simulink model "Ecotron"  (R2019b)
settings: Solver=FixedStepAuto  StartTime=0.0  StopTime=1  FixedStep=0.001  RelTol=1e-3  EnableMultiTasking=on
InitFcn:
  | EcoCoder_PreCheckLic();
libraries: CoderSF_BSW_Libs x228, SF_CanService_Libs x49, simulink x33, dspstat3 x6
(part 2 of 6)

== system Ecotron/Input/By-wire/Throttle Controller ==
  Bus Creator : BusCreator  Inputs=4
  Bus Creator1 : BusCreator  Inputs=4  OutDataTypeStr=Bus: Msg
      settings: InheritFromInputs=off
  Read CAN Message : SF_CanService_Libs/Read CAN Message  typeCAN=Connected  channel=CAN_C  mEn=off  msgInfo=Leo_accpedal  msgItermStore=Feedback  msgIterm=Feedback  valid=on  stale=on  motoBit=off  setSignalName=on  flgCustomMonitorVariableRules=on  defineSignalName=off  prefixSignal='rx'  flgValTest=off  flgNoFixed=on  tSample=Task_L1ms  modeCode=Parameterless
  Subsystem4 : Subsystem
  Write and Read Measurement : CoderSF_BSW_Libs/Calibration & Measurement/Write and Read Measurement  variable_name=THROTTLE_CurrentPedalPos  variable_value=0  variable_type=single  numD=1  unitStr=""  descStr=""
      settings: AttributesFormatString=type:%<variable_type> Dimensions:%<numD>  SourceProductName=EcoCoder Blocks
  Write and Read Measurement1 : CoderSF_BSW_Libs/Calibration & Measurement/Write and Read Measurement  variable_name=THROTTLE_ECUTimeout  variable_value=0  variable_type=single  numD=1  unitStr=""  descStr=""
      settings: AttributesFormatString=type:%<variable_type> Dimensions:%<numD>  SourceProductName=EcoCoder Blocks
  Write and Read Measurement2 : CoderSF_BSW_Libs/Calibration & Measurement/Write and Read Measurement  variable_name=THROTTLE_PedalConnectionError  variable_value=0  variable_type=single  numD=1  unitStr=""  descStr=""
      settings: AttributesFormatString=type:%<variable_type> Dimensions:%<numD>  SourceProductName=EcoCoder Blocks
  Throttle : Outport
  wires:
  Bus Creator/1 -> Throttle/1
  Read CAN Message/4 -> Write and Read Measurement1/1  "rxTimeout_Err"
  Read CAN Message/5 -> Write and Read Measurement2/1  "rxPedal_connErr"
  Subsystem4/2(Cnt) -> Bus Creator1/2  "Cnt"
  Subsystem4/4(Msg_Freq) -> Bus Creator1/4  "MsgFreq"
  Subsystem4/3(Timeout_Err) -> Bus Creator1/3  "Timeout"
  Subsystem4/1("Available ") -> Bus Creator1/1  "Available"
  Read CAN Message/1 -> Subsystem4/1("Available_in ")
  Read CAN Message/2 -> Subsystem4/2(Msg_cnt)
  Bus Creator1/1 -> Bus Creator/1  "Msg"
  Read CAN Message/3 -> Write and Read Measurement/1  "rxCurrent_PedalPos"
  Write and Read Measurement/1 -> Bus Creator/2  "THROTTLE_CurrentPedalPos"
  Write and Read Measurement1/1 -> Bus Creator/3  "THROTTLE_ECUTimeout"
  Write and Read Measurement2/1 -> Bus Creator/4  "THROTTLE_PedalConnectionError"

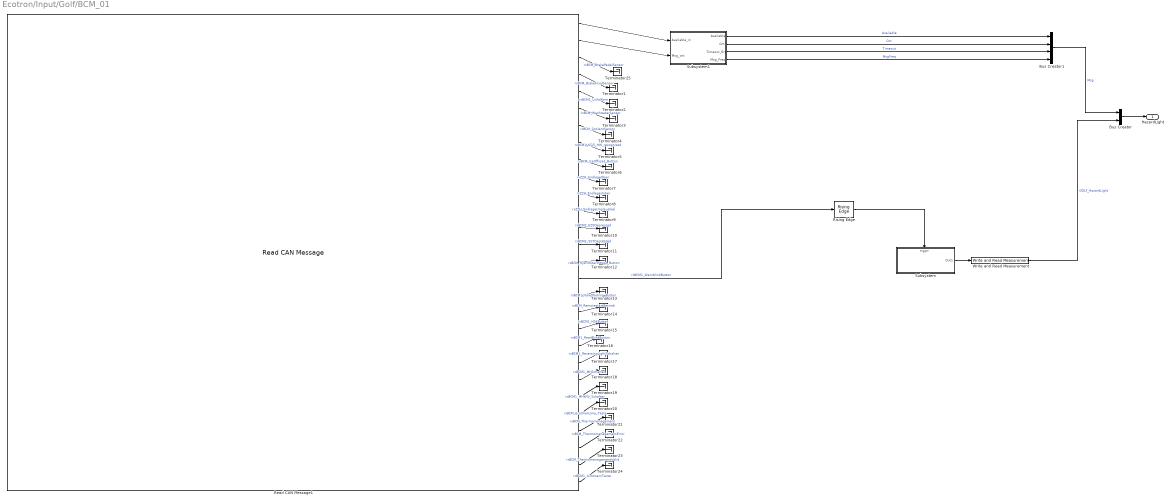
== system Ecotron/Input/Golf/BCM_01 ==
  Bus Creator : BusCreator  Inputs=2
  Bus Creator1 : BusCreator  Inputs=4  OutDataTypeStr=Bus: Msg
      settings: InheritFromInputs=off
  Read CAN Message1 : SF_CanService_Libs/Read CAN Message  typeCAN=Connected  channel=CAN_B  mEn=off  msgInfo=vw_golf  msgItermStore=BCM_01  msgIterm=BCM_01  valid=on  stale=on  motoBit=off  setSignalName=on  flgCustomMonitorVariableRules=on  defineSignalName=off  prefixSignal='rx'  flgValTest=off  flgNoFixed=on  tSample=Task_L1ms  modeCode=Parameterless
  Rising Edge : CoderSF_BSW_Libs/Application Base Blocks/Rising Edge  InitialCondition=off
      settings: SourceProductName=EcoCoder Blocks
  Subsystem : Subsystem
  Subsystem1 : Subsystem
  Terminator{1..25} (25 alike) : Terminator
  Write and Read Measurement : CoderSF_BSW_Libs/Calibration & Measurement/Write and Read Measurement  variable_name=GOLF_HazardLight  variable_value=0  variable_type=boolean  numD=1  unitStr=""  descStr=""
      settings: AttributesFormatString=type:%<variable_type> Dimensions:%<numD>  SourceProductName=EcoCoder Blocks
  HazardLight : Outport
  wires:
  Read CAN Message1/7 -> Terminator4/1  "rxBCM_CoolantSensor"
  Read CAN Message1/25 -> Terminator21/1  "rxBCM_Thermomanagement"
  Read CAN Message1/3 -> Terminator25/1  "rxBCM_BrakePedalSensor"
  Read CAN Message1/5 -> Terminator2/1  "rxBCM1_LichtWarn"
  Read CAN Message1/20 -> Terminator16/1  "rxBCM1_RearBlindButton"
  Read CAN Message1/4 -> Terminator1/1  "rxBCM_BrakeFluidSensor"
  Read CAN Message1/12 -> Terminator9/1  "rxZZH_EndlageUnplausibel"
  Read CAN Message1/11 -> Terminator8/1  "rxZZH_EndlageUnten"
  Read CAN Message1/9 -> Terminator6/1  "rxBCM_IceOffroad_Button"
  Read CAN Message1/28 -> Terminator24/1  "rxBCM1_LichtwarnTexte"
  Read CAN Message1/8 -> Terminator5/1  "rxBCM1_Kl15_HW_recognized"
  Read CAN Message1/6 -> Terminator3/1  "rxBCM_WashwaterSensor"
  Read CAN Message1/24 -> Terminator20/1  "rxBCM_EcoCharisma_Taste"
  Read CAN Message1/10 -> Terminator7/1  "rxZZH_EndlageOben"
  Read CAN Message1/14 -> Terminator11/1  "rxBCM2_SSTDepressed"
  Read CAN Message1/13 -> Terminator10/1  "rxBCM2_EZSDepressed"
  Read CAN Message1/15 -> Terminator12/1  "rxBCM_HybridStartStopp_Button"
  Read CAN Message1/17 -> Terminator13/1  "rxBCM1_ValetParking_Button"
  Read CAN Message1/18 -> Terminator14/1  "rxBCM_RemotestartBetrieb"
  Read CAN Message1/16 -> Rising Edge/1  "rxBCM1_WarnblinkButton"
  Read CAN Message1/22 -> Terminator18/1  "rxBCM1_MHSchalter"
  Read CAN Message1/19 -> Terminator15/1  "rxBCM1_HSKButton"
  Read CAN Message1/23 -> Terminator19/1  "rxBCM1_MHWIV_Schalter"
  Read CAN Message1/21 -> Terminator17/1  "rxBCM1_ReversingLightSchalter"
  Read CAN Message1/26 -> Terminator22/1  "rxBCM_ThermomanagementError"
  Read CAN Message1/27 -> Terminator23/1  "rxBCM_ThermomanagementValid"
  Subsystem1/2(Cnt) -> Bus Creator1/2  "Cnt"
  Subsystem1/1("Available ") -> Bus Creator1/1  "Available"
  Read CAN Message1/2 -> Subsystem1/2(Msg_cnt)
  Subsystem1/4(Msg_Freq) -> Bus Creator1/4  "MsgFreq"
  Bus Creator1/1 -> Bus Creator/1  "Msg"
  Read CAN Message1/1 -> Subsystem1/1("Available_in ")
  Subsystem1/3(Timeout_Err) -> Bus Creator1/3  "Timeout"
  Subsystem/1(Out1) -> Write and Read Measurement/1
  Rising Edge/1 -> Subsystem/Trigger
  Write and Read Measurement/1 -> Bus Creator/2  "GOLF_HazardLight"
  Bus Creator/1 -> HazardLight/1

== system Ecotron/Input/Golf/Brake ==
  Bus Creator : BusCreator  Inputs=2
  Bus Creator1 : BusCreator  Inputs=4  OutDataTypeStr=Bus: Msg
      settings: InheritFromInputs=off
  Read CAN Message : SF_CanService_Libs/Read CAN Message  typeCAN=Connected  channel=CAN_B  mEn=off  msgInfo=vw_golf  msgItermStore=Brake  msgIterm=Brake  valid=on  stale=on  motoBit=off  setSignalName=on  flgCustomMonitorVariableRules=on  defineSignalName=off  prefixSignal=''  flgValTest=off  flgNoFixed=on  tSample=Task_L1ms  modeCode=Parameterless
  Subsystem1 : Subsystem
  Write and Read Measurement : CoderSF_BSW_Libs/Calibration & Measurement/Write and Read Measurement  variable_name=GOLF_BrakePedalPos  variable_value=0  variable_type=single  numD=1  unitStr=""  descStr=""
      settings: AttributesFormatString=type:%<variable_type> Dimensions:%<numD>  SourceProductName=EcoCoder Blocks
  Brake : Outport
  wires:
  Subsystem1/2(Cnt) -> Bus Creator1/2  "Cnt"
  Subsystem1/4(Msg_Freq) -> Bus Creator1/4  "MsgFreq"
  Subsystem1/3(Timeout_Err) -> Bus Creator1/3  "Timeout"
  Subsystem1/1("Available ") -> Bus Creator1/1  "Available"
  Read CAN Message/1 -> Subsystem1/1("Available_in ")
  Read CAN Message/2 -> Subsystem1/2(Msg_cnt)
  Bus Creator1/1 -> Bus Creator/1  "Msg"
  Read CAN Message/3 -> Write and Read Measurement/1  "Brake_pedalPos"
  Bus Creator/1 -> Brake/1  "Brake"
  Write and Read Measurement/1 -> Bus Creator/2  "GOLF_BrakePedalPos"

== system Ecotron/Input/Golf/Brake and Steering Feedback Echo ==
  Receive CAN Message : CoderSF_BSW_Libs/CAN/Receive CAN Message  channel=CAN_B  txid=hex2dec('176')  extended=off  txlen=8  tasktimeIndex=Task_L1ms
      settings: SourceProductName=EcoCoder Blocks
  Receive CAN Message1 : CoderSF_BSW_Libs/CAN/Receive CAN Message  channel=CAN_B  txid=hex2dec('86')  extended=off  txlen=8  tasktimeIndex=Task_L1ms
      settings: SourceProductName=EcoCoder Blocks
  Subsystem2 : Subsystem
  Subsystem7 : Subsystem
  Terminator{2..9} (8 alike) : Terminator
  wires:
  Receive CAN Message/4 -> Terminator5/1
  Receive CAN Message1/3 -> Terminator8/1
  Receive CAN Message1/4 -> Terminator3/1
  Receive CAN Message/6 -> Subsystem2/1(In1)
  Receive CAN Message1/5 -> Terminator2/1
  Receive CAN Message1/2 -> Terminator9/1
  Receive CAN Message/3 -> Terminator6/1
  Receive CAN Message1/6 -> Subsystem7/1(In1)
  Receive CAN Message1/1 -> Subsystem7/Trigger
  Receive CAN Message/5 -> Terminator4/1
  Receive CAN Message/1 -> Subsystem2/Trigger
  Receive CAN Message/2 -> Terminator7/1

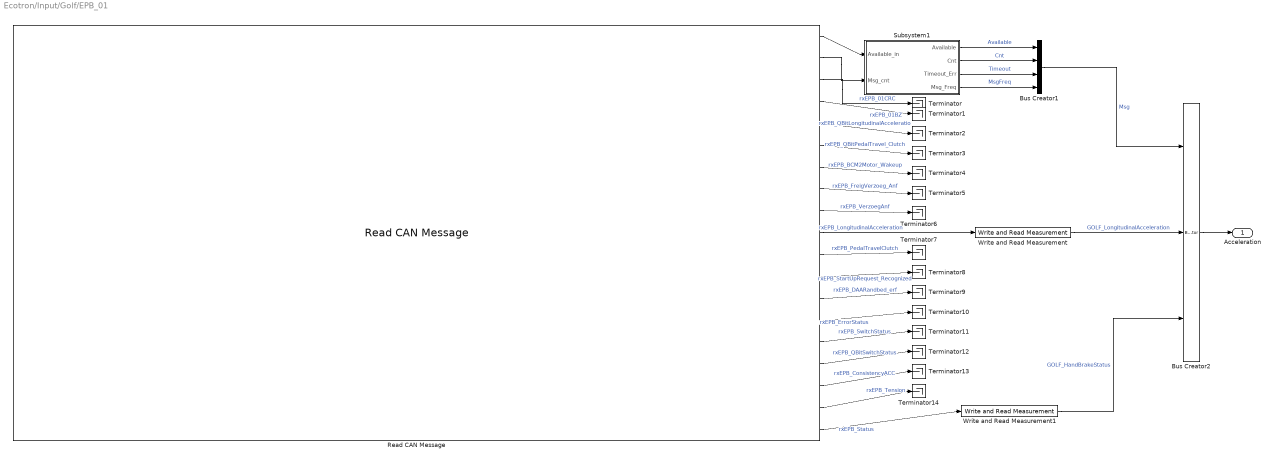
== system Ecotron/Input/Golf/EPB_01 ==
  Bus Creator1 : BusCreator  Inputs=4  OutDataTypeStr=Bus: Msg
      settings: InheritFromInputs=off
  Bus Creator2 : BusCreator  Inputs=3
  Read CAN Message : SF_CanService_Libs/Read CAN Message  typeCAN=Connected  channel=CAN_B  mEn=off  msgInfo=vw_golf  msgItermStore=EPB_01  msgIterm=EPB_01  valid=on  stale=on  motoBit=off  setSignalName=on  flgCustomMonitorVariableRules=on  defineSignalName=off  prefixSignal='rx'  flgValTest=off  flgNoFixed=on  tSample=Task_L1ms  modeCode=Parameterless
  Subsystem1 : Subsystem
  Terminator{,1..14} (15 alike) : Terminator
  Write and Read Measurement : CoderSF_BSW_Libs/Calibration & Measurement/Write and Read Measurement  variable_name=GOLF_LongitudinalAcceleration  variable_value=0  variable_type=single  numD=1  unitStr=""  descStr=""
      settings: AttributesFormatString=type:%<variable_type> Dimensions:%<numD>  SourceProductName=EcoCoder Blocks
  Write and Read Measurement1 : CoderSF_BSW_Libs/Calibration & Measurement/Write and Read Measurement  variable_name=GOLF_HandBrakeStatus  variable_value=0  variable_type=single  numD=1  unitStr=""  descStr=""
      settings: AttributesFormatString=type:%<variable_type> Dimensions:%<numD>  SourceProductName=EcoCoder Blocks
  Acceleration : Outport
  wires:
  Read CAN Message/8 -> Terminator5/1  "rxEPB_FreigVerzoeg_Anf"
  Read CAN Message/6 -> Terminator3/1  "rxEPB_QBitPedalTravel_Clutch"
  Subsystem1/2(Cnt) -> Bus Creator1/2  "Cnt"
  Subsystem1/1("Available ") -> Bus Creator1/1  "Available"
  Read CAN Message/19 -> Write and Read Measurement1/1  "rxEPB_Status"
  Read CAN Message/3 -> Terminator/1  "rxEPB_01CRC"
  Read CAN Message/2 -> Subsystem1/2(Msg_cnt)
  Read CAN Message/11 -> Terminator7/1  "rxEPB_PedalTravelClutch"
  Read CAN Message/16 -> Terminator12/1  "rxEPB_QBitSwitchStatus"
  Read CAN Message/7 -> Terminator4/1  "rxEPB_BCM2Motor_Wakeup"
  Read CAN Message/14 -> Terminator10/1  "rxEPB_ErrorStatus"
  Read CAN Message/9 -> Terminator6/1  "rxEPB_VerzoegAnf"
  Subsystem1/4(Msg_Freq) -> Bus Creator1/4  "MsgFreq"
  Read CAN Message/15 -> Terminator11/1  "rxEPB_SwitchStatus"
  Subsystem1/3(Timeout_Err) -> Bus Creator1/3  "Timeout"
  Read CAN Message/13 -> Terminator9/1  "rxEPB_DAARandbed_erf"
  Read CAN Message/4 -> Terminator1/1  "rxEPB_01BZ"
  Read CAN Message/10 -> Write and Read Measurement/1  "rxEPB_LongitudinalAcceleration"
  Read CAN Message/18 -> Terminator14/1  "rxEPB_Tension"
  Read CAN Message/5 -> Terminator2/1  "rxEPB_QBitLongitudinalAcceleratio"
  Read CAN Message/12 -> Terminator8/1  "rxEPB_StartUpRequest_Recognized"
  Read CAN Message/1 -> Subsystem1/1("Available_in ")
  Bus Creator1/1 -> Bus Creator2/1  "Msg"
  Read CAN Message/17 -> Terminator13/1  "rxEPB_ConsistencyACC"
  Bus Creator2/1 -> Acceleration/1
  Write and Read Measurement/1 -> Bus Creator2/2  "GOLF_LongitudinalAcceleration"
  Write and Read Measurement1/1 -> Bus Creator2/3  "GOLF_HandBrakeStatus"

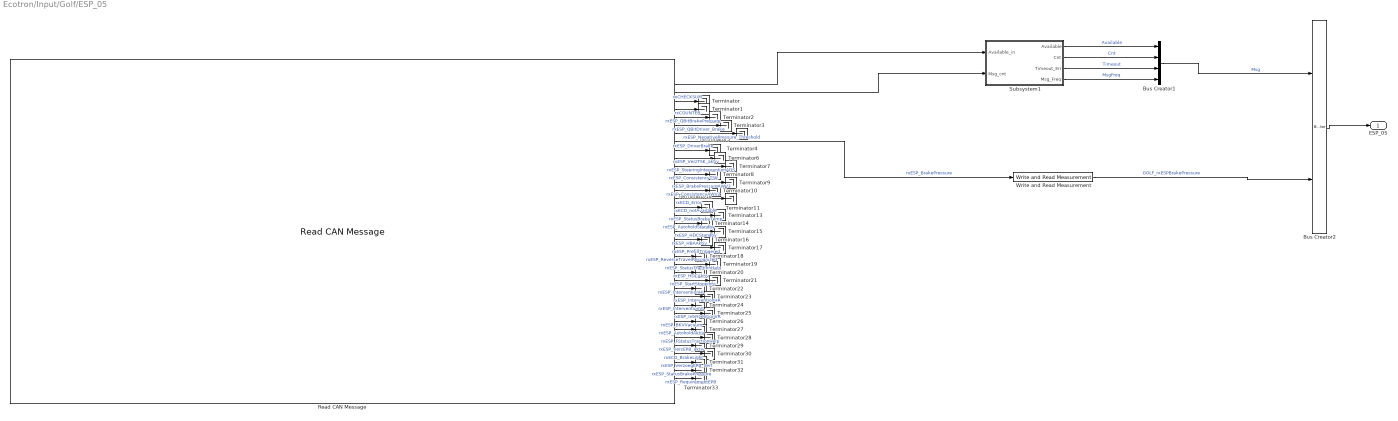
== system Ecotron/Input/Golf/ESP_05 ==
  Bus Creator1 : BusCreator  Inputs=4  OutDataTypeStr=Bus: Msg
      settings: InheritFromInputs=off
  Bus Creator2 : BusCreator  Inputs=2
  Read CAN Message : SF_CanService_Libs/Read CAN Message  typeCAN=Connected  channel=CAN_B  mEn=off  msgInfo=vw_golf  msgItermStore=ESP_05  msgIterm=ESP_05  valid=on  stale=on  motoBit=off  setSignalName=on  flgCustomMonitorVariableRules=on  defineSignalName=off  prefixSignal='rx'  flgValTest=off  flgNoFixed=on  tSample=Task_L1ms  modeCode=Parameterless
  Subsystem1 : Subsystem
  Terminator{,1..33} (34 alike) : Terminator
  Write and Read Measurement : CoderSF_BSW_Libs/Calibration & Measurement/Write and Read Measurement  variable_name=GOLF_rxESPBrakePressure  variable_value=0  variable_type=single  numD=1  unitStr=""  descStr=""
      settings: AttributesFormatString=type:%<variable_type> Dimensions:%<numD>  SourceProductName=EcoCoder Blocks
  ESP_05 : Outport
  wires:
  Subsystem1/1("Available ") -> Bus Creator1/1  "Available"
  Bus Creator2/1 -> ESP_05/1
  Read CAN Message/2 -> Subsystem1/2(Msg_cnt)
  Subsystem1/2(Cnt) -> Bus Creator1/2  "Cnt"
  Read CAN Message/1 -> Subsystem1/1("Available_in ")
  Subsystem1/3(Timeout_Err) -> Bus Creator1/3  "Timeout"
  Bus Creator1/1 -> Bus Creator2/1  "Msg"
  Subsystem1/4(Msg_Freq) -> Bus Creator1/4  "MsgFreq"
  Write and Read Measurement/1 -> Bus Creator2/2  "GOLF_rxESPBrakePressure"
  Read CAN Message/8 -> Write and Read Measurement/1  "rxESP_BrakePressure"
  Read CAN Message/3 -> Terminator/1  "rxCHECKSUM"
  Read CAN Message/4 -> Terminator1/1  "rxCOUNTER"
  Read CAN Message/5 -> Terminator2/1  "rxESP_QBitBrakePressure"
  Read CAN Message/6 -> Terminator3/1  "rxESP_QBitDriver_Brake"
  Read CAN Message/7 -> Terminator4/1  "rxESP_NegativePressure_Threshold"
  Read CAN Message/9 -> Terminator5/1  "rxESP_DriverBrake"
  Read CAN Message/10 -> Terminator6/1  "rxESP_VerzTSK_aktiv"
  Read CAN Message/11 -> Terminator7/1  "rxESP_SteeringInterventionADS"
  Read CAN Message/12 -> Terminator8/1  "rxESP_ConsistencyTSK"
  Read CAN Message/13 -> Terminator9/1  "rxESP_BrakePressureAWV2"
  Read CAN Message/14 -> Terminator10/1  "rxESP_ConsistencyAWV2"
  Read CAN Message/15 -> Terminator11/1  "rxECD_Error"
  Read CAN Message/16 -> Terminator12/1  "rxECD_notAvailable"
  Read CAN Message/17 -> Terminator13/1  "rxESP_StatusBrakeTemp"
  Read CAN Message/18 -> Terminator14/1  "rxESP_AutoholdStandby"
  Read CAN Message/19 -> Terminator15/1  "rxESP_HDCStandby"
  Read CAN Message/20 -> Terminator16/1  "rxESP_HBAAktiv"
  Read CAN Message/21 -> Terminator17/1  "rxESP_PrefillTriggered"
  Read CAN Message/22 -> Terminator18/1  "rxESP_ReverseTravelRecognized"
  Read CAN Message/23 -> Terminator19/1  "rxESP_StatusTractionHelp"
  Read CAN Message/24 -> Terminator20/1  "rxESP_HDCAktiv"
  Read CAN Message/25 -> Terminator21/1  "rxESP_StartStoppInfo"
  Read CAN Message/26 -> Terminator22/1  "rxESP_InterventionHL"
  Read CAN Message/27 -> Terminator23/1  "rxESP_InterventionHR"
  Read CAN Message/28 -> Terminator24/1  "rxESP_InterventionVL"
  Read CAN Message/29 -> Terminator25/1  "rxESP_InterventionVR"
  Read CAN Message/30 -> Terminator26/1  "rxESP_BKVVacuum"
  Read CAN Message/31 -> Terminator27/1  "rxESP_AutoholdAktiv"
  Read CAN Message/32 -> Terminator28/1  "rxESP_FStatusTractionHelp"
  Read CAN Message/33 -> Terminator29/1  "rxESP_VerzEPB_aktiv"
  Read CAN Message/34 -> Terminator30/1  "rxECD_BrakeLight"
  Read CAN Message/35 -> Terminator31/1  "rxESP_VerzoegEPB_verf"
  Read CAN Message/36 -> Terminator32/1  "rxESP_StatusBrakePressure"
  Read CAN Message/37 -> Terminator33/1  "rxESP_RequirementEPB"

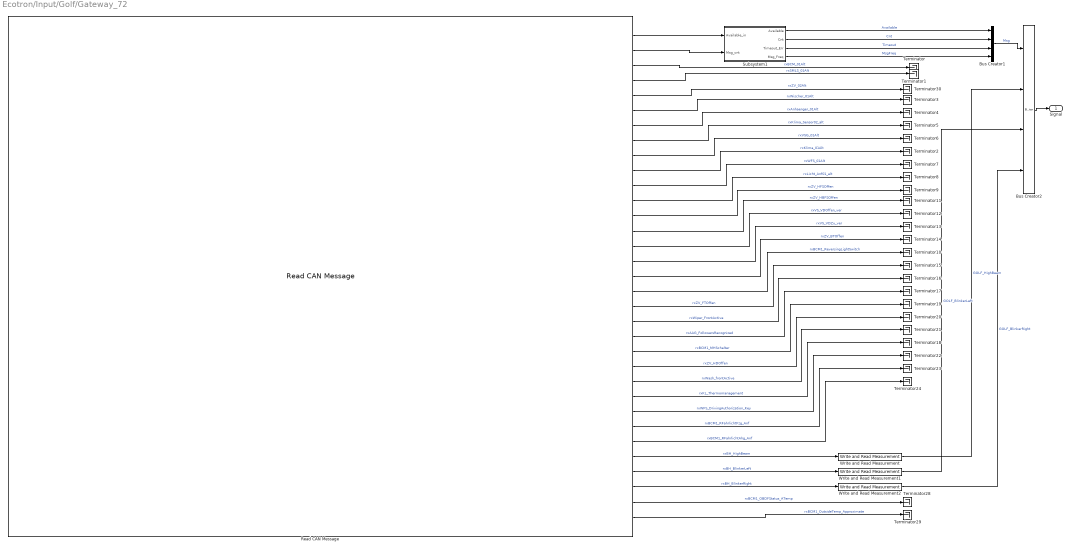
== system Ecotron/Input/Golf/Gateway_72 ==
  Bus Creator1 : BusCreator  Inputs=4  OutDataTypeStr=Bus: Msg
      settings: InheritFromInputs=off
  Bus Creator2 : BusCreator  Inputs=4
  Read CAN Message : SF_CanService_Libs/Read CAN Message  typeCAN=Connected  channel=CAN_B  mEn=off  msgInfo=vw_golf  msgItermStore=Gateway_72  msgIterm=Gateway_72  valid=on  stale=on  motoBit=off  setSignalName=on  flgCustomMonitorVariableRules=on  defineSignalName=off  prefixSignal='rx'  flgValTest=off  flgNoFixed=on  tSample=Task_L1ms  modeCode=Parameterless
  Subsystem1 : Subsystem
  Terminator{,1..24,28..30} (28 alike) : Terminator
  Write and Read Measurement : CoderSF_BSW_Libs/Calibration & Measurement/Write and Read Measurement  variable_name=GOLF_HighBeam  variable_value=0  variable_type=single  numD=1  unitStr=""  descStr=""
      settings: AttributesFormatString=type:%<variable_type> Dimensions:%<numD>  SourceProductName=EcoCoder Blocks
  Write and Read Measurement1 : CoderSF_BSW_Libs/Calibration & Measurement/Write and Read Measurement  variable_name=GOLF_BlinkerLeft  variable_value=0  variable_type=single  numD=1  unitStr=""  descStr=""
      settings: AttributesFormatString=type:%<variable_type> Dimensions:%<numD>  SourceProductName=EcoCoder Blocks
  Write and Read Measurement2 : CoderSF_BSW_Libs/Calibration & Measurement/Write and Read Measurement  variable_name=GOLF_BlinkerRight  variable_value=0  variable_type=single  numD=1  unitStr=""  descStr=""
      settings: AttributesFormatString=type:%<variable_type> Dimensions:%<numD>  SourceProductName=EcoCoder Blocks
  Signal : Outport
  wires:
  Read CAN Message/33 -> Terminator29/1  "rxBCM1_OutsideTemp_Approximate"
  Read CAN Message/32 -> Terminator28/1  "rxBCM1_OBDFStatus_ATemp"
  Read CAN Message/28 -> Terminator24/1  "rxBCM1_RFahrlichtAhg_Anf"
  Read CAN Message/27 -> Terminator23/1  "rxBCM1_RFahrlichtFzg_Anf"
  Read CAN Message/26 -> Terminator22/1  "rxWFS_DrivingAuthorization_Key"
  Read CAN Message/25 -> Terminator18/1  "rxKL_Thermomanagement"
  Read CAN Message/24 -> Terminator21/1  "rxWash_frontActive"
  Read CAN Message/23 -> Terminator20/1  "rxZV_HDOffen"
  Read CAN Message/22 -> Terminator19/1  "rxBCM1_MHSchalter"
  Read CAN Message/21 -> Terminator17/1  "rxAAG_FollowersRecognized"
  Read CAN Message/20 -> Terminator16/1  "rxWiper_FrontActive"
  Read CAN Message/19 -> Terminator15/1  "rxZV_FTOffen"
  Read CAN Message/18 -> Terminator10/1  "rxBCM1_ReversingLightSwitch"
  Read CAN Message/17 -> Terminator14/1  "rxZV_BTOffen"
  Read CAN Message/16 -> Terminator13/1  "rxVS_VDZu_ver"
  Read CAN Message/15 -> Terminator12/1  "rxVS_VDOffen_ver"
  Read CAN Message/14 -> Terminator11/1  "rxZV_HBFSOffen"
  Read CAN Message/12 -> Terminator8/1  "rxLicht_Anf01_alt"
  Subsystem1/4(Msg_Freq) -> Bus Creator1/4  "MsgFreq"
  Read CAN Message/4 -> Terminator1/1  "rxSMLS_01Alt"
  Read CAN Message/8 -> Terminator5/1  "rxKlima_Sensor02_alt"
  Read CAN Message/13 -> Terminator9/1  "rxZV_HFSOffen"
  Bus Creator1/1 -> Bus Creator2/1  "Msg"
  Subsystem1/3(Timeout_Err) -> Bus Creator1/3  "Timeout"
  Read CAN Message/9 -> Terminator6/1  "rxVSG_01Alt"
  Read CAN Message/1 -> Subsystem1/1("Available_in ")
  Read CAN Message/10 -> Terminator2/1  "rxKlima_01Alt"
  Read CAN Message/6 -> Terminator3/1  "rxWischer_01Alt"
  Read CAN Message/11 -> Terminator7/1  "rxWFS_01Alt"
  Read CAN Message/3 -> Terminator/1  "rxBCM_01Alt"
  Subsystem1/2(Cnt) -> Bus Creator1/2  "Cnt"
  Read CAN Message/7 -> Terminator4/1  "rxAnhaenger_01Alt"
  Read CAN Message/2 -> Subsystem1/2(Msg_cnt)
  Bus Creator2/1 -> Signal/1
  Subsystem1/1("Available ") -> Bus Creator1/1  "Available"
  Read CAN Message/5 -> Terminator30/1  "rxZV_02Alt"
  Read CAN Message/29 -> Write and Read Measurement/1  "rxBH_HighBeam"
  Read CAN Message/30 -> Write and Read Measurement1/1  "rxBH_BlinkerLeft"
  Read CAN Message/31 -> Write and Read Measurement2/1  "rxBH_BlinkerRight"
  Write and Read Measurement/1 -> Bus Creator2/2  "GOLF_HighBeam"
  Write and Read Measurement1/1 -> Bus Creator2/3  "GOLF_BlinkerLeft"
  Write and Read Measurement2/1 -> Bus Creator2/4  "GOLF_BlinkerRight"

== system Ecotron/Input/Golf/Getriebe_1 ==
  Bus Creator1 : BusCreator  Inputs=4  OutDataTypeStr=Bus: Msg
      settings: InheritFromInputs=off
  Bus Creator2 : BusCreator  Inputs=2
  Read CAN Message : SF_CanService_Libs/Read CAN Message  typeCAN=Connected  channel=CAN_B  mEn=off  msgInfo=vw_golf  msgItermStore=ESP_02  msgIterm=ESP_02  valid=on  stale=on  motoBit=off  setSignalName=on  flgCustomMonitorVariableRules=on  defineSignalName=off  prefixSignal='rx'  flgValTest=off  flgNoFixed=on  tSample=Task_L1ms  modeCode=Parameterless
  Subsystem1 : Subsystem
  Terminator{,1,3..15} (15 alike) : Terminator
  Write and Read Measurement : CoderSF_BSW_Libs/Calibration & Measurement/Write and Read Measurement  variable_name=GOLF_rxACC  variable_value=0  variable_type=single  numD=1  unitStr=""  descStr=""
      settings: AttributesFormatString=type:%<variable_type> Dimensions:%<numD>  SourceProductName=EcoCoder Blocks
  ACC : Outport
  wires:
  Read CAN Message/13 -> Terminator10/1  "rxESP_YawRate"
  Read CAN Message/5 -> Terminator9/1  "rxESP_QBitYawRate"
  Subsystem1/1("Available ") -> Bus Creator1/1  "Available"
  Bus Creator2/1 -> ACC/1
  Read CAN Message/2 -> Subsystem1/2(Msg_cnt)
  Subsystem1/2(Cnt) -> Bus Creator1/2  "Cnt"
  Read CAN Message/1 -> Subsystem1/1("Available_in ")
  Subsystem1/3(Timeout_Err) -> Bus Creator1/3  "Timeout"
  Bus Creator1/1 -> Bus Creator2/1  "Msg"
  Subsystem1/4(Msg_Freq) -> Bus Creator1/4  "MsgFreq"
  Read CAN Message/9 -> Terminator6/1  "rxESP_LateralAcceleration"
  Read CAN Message/8 -> Terminator5/1  "rxESP_Standstillflag"
  Read CAN Message/7 -> Terminator4/1  "rxESP_QBitLateral"
  Read CAN Message/6 -> Terminator3/1  "rxESP_QBitLongitudinalAcceleratio"
  Read CAN Message/4 -> Terminator1/1  "rxESP_02BZ"
  Read CAN Message/3 -> Terminator/1  "rxESP_02CRC"
  Write and Read Measurement/1 -> Bus Creator2/2  "GOLF_rxACC"
  Read CAN Message/12 -> Terminator8/1  "rxESP_QBitAnf_Vert_Wank"
  Read CAN Message/11 -> Terminator7/1  "rxESP_VerteilWankmom"
  Read CAN Message/10 -> Write and Read Measurement/1  "rxESP_LongitudinalAcceleration"
  Read CAN Message/18 -> Terminator15/1  "rxESP_StatusESP_PLA"
  Read CAN Message/17 -> Terminator14/1  "rxESP_PLACancellation"
  Read CAN Message/14 -> Terminator11/1  "rxESP_VZYawRate"
  Read CAN Message/15 -> Terminator12/1  "rxESP_EmergencyBrakeIndicator"
  Read CAN Message/16 -> Terminator13/1  "rxESP_StartVoltage"

== system Ecotron/Input/Golf/Getriebe_11 ==
  Bus Creator1 : BusCreator  Inputs=4  OutDataTypeStr=Bus: Msg
      settings: InheritFromInputs=off
  Bus Creator2 : BusCreator  Inputs=2
  Delay : Delay  DelayLength=7  UseCircularBuffer=on  SampleTime=0.1
  Read CAN Message : SF_CanService_Libs/Read CAN Message  typeCAN=Connected  channel=CAN_B  mEn=off  msgInfo=vw_golf  msgItermStore=Getriebe_11  msgIterm=Getriebe_11  valid=on  stale=on  motoBit=off  setSignalName=on  flgCustomMonitorVariableRules=on  defineSignalName=off  prefixSignal='rx'  flgValTest=off  flgNoFixed=on  tSample=Task_L1ms  modeCode=Parameterless
  Subsystem1 : Subsystem
  Terminator{,1..10} (11 alike) : Terminator
  Write and Read Measurement : CoderSF_BSW_Libs/Calibration & Measurement/Write and Read Measurement  variable_name=GOLF_GearLevel  variable_value=0  variable_type=single  numD=1  unitStr=""  descStr=""
      settings: AttributesFormatString=type:%<variable_type> Dimensions:%<numD>  SourceProductName=EcoCoder Blocks
  GearLevel : Outport
  wires:
  Read CAN Message/10 -> Terminator2/1  "rxGE_StatusCoupling"
  Read CAN Message/11 -> Terminator7/1  "rxGE_MMomStatus"
  Read CAN Message/12 -> Terminator8/1  "rxGE_ReleasedMMom_Hold"
  Write and Read Measurement/1 -> Bus Creator2/2  "GOLF_GearLevel"
  Read CAN Message/3 -> Terminator/1  "rxCHECKSUM"
  Read CAN Message/4 -> Terminator1/1  "rxCOUNTERXX"
  Read CAN Message/6 -> Terminator3/1  "rxGE_MMomHold_02"
  Read CAN Message/7 -> Terminator4/1  "rxGE_Uefkt"
  Read CAN Message/8 -> Terminator5/1  "rxGE_SpeedLevel"
  Read CAN Message/9 -> Terminator6/1  "rxGE_SwitchingProcess"
  Subsystem1/4(Msg_Freq) -> Bus Creator1/4  "MsgFreq"
  Bus Creator1/1 -> Bus Creator2/1  "Msg"
  Subsystem1/3(Timeout_Err) -> Bus Creator1/3  "Timeout"
  Read CAN Message/1 -> Subsystem1/1("Available_in ")
  Subsystem1/2(Cnt) -> Bus Creator1/2  "Cnt"
  Read CAN Message/2 -> Subsystem1/2(Msg_cnt)
  Bus Creator2/1 -> GearLevel/1
  Subsystem1/1("Available ") -> Bus Creator1/1  "Available"
  Read CAN Message/14 -> Delay/1  "rxGE_TargetWalk"
  Read CAN Message/5 -> Terminator9/1  "rxGE_MMomSoll_02"
  Read CAN Message/13 -> Terminator10/1  "rxGE_BanFadingOut"
  Delay/1 -> Write and Read Measurement/1

== system Ecotron/Input/Golf/Getriebe_2 ==
  Bus Creator1 : BusCreator  Inputs=4  OutDataTypeStr=Bus: Msg
      settings: InheritFromInputs=off
  Bus Creator2 : BusCreator  Inputs=3
  Read CAN Message : SF_CanService_Libs/Read CAN Message  typeCAN=Connected  channel=CAN_B  mEn=off  msgInfo=vw_golf  msgItermStore=Motor_16  msgIterm=Motor_16  valid=on  stale=on  motoBit=off  setSignalName=on  flgCustomMonitorVariableRules=on  defineSignalName=off  prefixSignal='rx'  flgValTest=off  flgNoFixed=on  tSample=Task_L1ms  modeCode=Parameterless
  Subsystem1 : Subsystem
  Terminator{,1..5} (6 alike) : Terminator
  Write and Read Measurement : CoderSF_BSW_Libs/Calibration & Measurement/Write and Read Measurement  variable_name=GOLF_rxVehiclemass  variable_value=0  variable_type=uint32  numD=1  unitStr=""  descStr=""
      settings: AttributesFormatString=type:%<variable_type> Dimensions:%<numD>  SourceProductName=EcoCoder Blocks
  Write and Read Measurement1 : CoderSF_BSW_Libs/Calibration & Measurement/Write and Read Measurement  variable_name=GOLF_rxPitch  variable_value=0  variable_type=single  numD=1  unitStr=""  descStr=""
      settings: AttributesFormatString=type:%<variable_type> Dimensions:%<numD>  SourceProductName=EcoCoder Blocks
  TSK : Outport
  wires:
  Write and Read Measurement/1 -> Bus Creator2/2  "GOLF_rxVehiclemass"
  Subsystem1/4(Msg_Freq) -> Bus Creator1/4  "MsgFreq"
  Bus Creator1/1 -> Bus Creator2/1  "Msg"
  Subsystem1/3(Timeout_Err) -> Bus Creator1/3  "Timeout"
  Read CAN Message/1 -> Subsystem1/1("Available_in ")
  Subsystem1/2(Cnt) -> Bus Creator1/2  "Cnt"
  Read CAN Message/2 -> Subsystem1/2(Msg_cnt)
  Bus Creator2/1 -> TSK/1
  Subsystem1/1("Available ") -> Bus Creator1/1  "Available"
  Read CAN Message/9 -> Write and Read Measurement/1  "rxTSK_VehicleMass02"
  Read CAN Message/10 -> Write and Read Measurement1/1  "rxTSK_Pitch"
  Write and Read Measurement1/1 -> Bus Creator2/3  "GOLF_rxPitch"
  Read CAN Message/3 -> Terminator/1  "rxTSK_QBitPitch"
  Read CAN Message/4 -> Terminator1/1  "rxTSK_QBitVehicleMass"
  Read CAN Message/5 -> Terminator2/1  "rxMO_StartVoltage02"
  Read CAN Message/6 -> Terminator3/1  "rxMO_DPFReg"
  Read CAN Message/7 -> Terminator4/1  "rxMO_HeaetingcurrentEKAT"
  Read CAN Message/8 -> Terminator5/1  "rxMO_HeaetingcurrentSCR"

== system Ecotron/Input/Golf/Kombi_02 ==
  Bus Creator : BusCreator  Inputs=3
  Bus Creator1 : BusCreator  Inputs=4  OutDataTypeStr=Bus: Msg
      settings: InheritFromInputs=off
  Constant : Constant  Value=50
  Divide : Product  Inputs=*/  OutDataTypeStr=single
  Read CAN Message1 : SF_CanService_Libs/Read CAN Message  typeCAN=Connected  channel=CAN_B  mEn=off  msgInfo=vw_golf  msgItermStore=Kombi_02  msgIterm=Kombi_02  valid=on  stale=on  motoBit=off  setSignalName=on  flgCustomMonitorVariableRules=on  defineSignalName=off  prefixSignal='rx'  flgValTest=off  flgNoFixed=on  tSample=Task_L1ms  modeCode=Parameterless
  Subsystem1 : Subsystem
  Terminator{,1..4} (5 alike) : Terminator
  Write and Read Measurement : CoderSF_BSW_Libs/Calibration & Measurement/Write and Read Measurement  variable_name=GOLF_Fuel  variable_value=0  variable_type=single  numD=1  unitStr=liter  descStr=""
      settings: AttributesFormatString=type:%<variable_type> Dimensions:%<numD>  SourceProductName=EcoCoder Blocks
  Write and Read Measurement1 : CoderSF_BSW_Libs/Calibration & Measurement/Write and Read Measurement  variable_name=GOLF_Fuel_ratio  variable_value=0  variable_type=single  numD=1  unitStr=liter  descStr=""
      settings: AttributesFormatString=type:%<variable_type> Dimensions:%<numD>  SourceProductName=EcoCoder Blocks
  Fuel_Tank : Outport
  wires:
  Bus Creator/1 -> Fuel_Tank/1
  Subsystem1/3(Timeout_Err) -> Bus Creator1/3  "Timeout"
  Read CAN Message1/1 -> Subsystem1/1("Available_in ")
  Bus Creator1/1 -> Bus Creator/1  "Msg"
  Subsystem1/4(Msg_Freq) -> Bus Creator1/4  "MsgFreq"
  Read CAN Message1/2 -> Subsystem1/2(Msg_cnt)
  Subsystem1/1("Available ") -> Bus Creator1/1  "Available"
  Subsystem1/2(Cnt) -> Bus Creator1/2  "Cnt"
  Read CAN Message1/5 -> Divide/1, Write and Read Measurement/1  "rxKBI_InhaltTank"
  Write and Read Measurement/1 -> Bus Creator/2  "GOLF_Fuel"
  Constant/1 -> Divide/2
  Divide/1 -> Write and Read Measurement1/1
  Write and Read Measurement1/1 -> Bus Creator/3  "GOLF_Fuel_ratio"
  Read CAN Message1/4 -> Terminator/1  "rxKBI_Standzeit02"
  Read CAN Message1/3 -> Terminator1/1  "rxKBI_Kilometerstand"
  Read CAN Message1/6 -> Terminator2/1  "rxKBI_FStatusTank"
  Read CAN Message1/7 -> Terminator3/1  "rxKBI_QBitAussen_Temp_gef"
  Read CAN Message1/8 -> Terminator4/1  "rxKBI_AussenTemp_gef"

== system Ecotron/Input/Golf/LWl ==
  Bus Creator : BusCreator  Inputs=11
  Bus Creator1 : BusCreator  Inputs=4  OutDataTypeStr=Bus: Msg
      settings: InheritFromInputs=off
  Bus Creator2 : BusCreator  Inputs=3
  Bus Selector : BusSelector  OutputSignals=GOLF_LWIVZ_SteeringWheelAngle,GOLF_LWI_SteeringWheelAngle,GOLF_LWIVZ_SteeringWheelAngle_Speed,GOLF_LWI_SteeringWheelAngle_Speed
  Constant : Constant
  Constant1 : Constant  Value=-1
  Constant2 : Constant
  Constant3 : Constant  Value=-1
  Product : Product
  Product1 : Product
  Read CAN Message : SF_CanService_Libs/Read CAN Message  typeCAN=Connected  channel=CAN_B  mEn=off  msgInfo=vw_golf  msgItermStore=LWI_01  msgIterm=LWI_01  valid=on  stale=on  motoBit=off  setSignalName=on  flgCustomMonitorVariableRules=on  defineSignalName=off  prefixSignal='LWI_'  flgValTest=off  flgNoFixed=on  tSample=Task_L1ms  modeCode=Parameterless
  Subsystem1 : Subsystem
  Switch : Switch  Criteria=u2 > Threshold  Threshold=0.5  OutDataTypeStr=single
  Switch1 : Switch  Criteria=u2 > Threshold  Threshold=0.5  OutDataTypeStr=single
  Write and Read Measurement : CoderSF_BSW_Libs/Calibration & Measurement/Write and Read Measurement  variable_name=GOLF_LWIQbit_SteeringWheelAngle  variable_value=0  variable_type=single  numD=1  unitStr=""  descStr=""
      settings: AttributesFormatString=type:%<variable_type> Dimensions:%<numD>  SourceProductName=EcoCoder Blocks
  Write and Read Measurement1 : CoderSF_BSW_Libs/Calibration & Measurement/Write and Read Measurement  variable_name=GOLF_LWI_SteeringWheelAngle  variable_value=0  variable_type=single  numD=1  unitStr=""  descStr=""
      settings: AttributesFormatString=type:%<variable_type> Dimensions:%<numD>  SourceProductName=EcoCoder Blocks
  Write and Read Measurement2 : CoderSF_BSW_Libs/Calibration & Measurement/Write and Read Measurement  variable_name=GOLF_LWIVZ_SteeringWheelAngle  variable_value=0  variable_type=single  numD=1  unitStr=""  descStr=""
      settings: AttributesFormatString=type:%<variable_type> Dimensions:%<numD>  SourceProductName=EcoCoder Blocks
  Write and Read Measurement3 : CoderSF_BSW_Libs/Calibration & Measurement/Write and Read Measurement  variable_name=GOLF_LWIVZ_SteeringWheelAngle_Speed  variable_value=0  variable_type=single  numD=1  unitStr=""  descStr=""
      settings: AttributesFormatString=type:%<variable_type> Dimensions:%<numD>  SourceProductName=EcoCoder Blocks
  Write and Read Measurement4 : CoderSF_BSW_Libs/Calibration & Measurement/Write and Read Measurement  variable_name=GOLF_LWI_SteeringWheelAngle_Speed  variable_value=0  variable_type=single  numD=1  unitStr=""  descStr=""
      settings: AttributesFormatString=type:%<variable_type> Dimensions:%<numD>  SourceProductName=EcoCoder Blocks
  Write and Read Measurement5 : CoderSF_BSW_Libs/Calibration & Measurement/Write and Read Measurement  variable_name=Steering_Angle  variable_value=0  variable_type=single  numD=1  unitStr=""  descStr=""
      settings: AttributesFormatString=type:%<variable_type> Dimensions:%<numD>  SourceProductName=EcoCoder Blocks
  Write and Read Measurement6 : CoderSF_BSW_Libs/Calibration & Measurement/Write and Read Measurement  variable_name=Steering_Angle_Speed  variable_value=0  variable_type=single  numD=1  unitStr=""  descStr=""
      settings: AttributesFormatString=type:%<variable_type> Dimensions:%<numD>  SourceProductName=EcoCoder Blocks
  LWI : Outport
  wires:
  Subsystem1/2(Cnt) -> Bus Creator1/2  "Cnt"
  Subsystem1/4(Msg_Freq) -> Bus Creator1/4  "MsgFreq"
  Subsystem1/3(Timeout_Err) -> Bus Creator1/3  "Timeout"
  Subsystem1/1("Available ") -> Bus Creator1/1  "Available"
  Read CAN Message/1 -> Subsystem1/1("Available_in ")
  Read CAN Message/2 -> Subsystem1/2(Msg_cnt)
  Bus Creator1/1 -> Bus Creator/1  "Msg"
  Read CAN Message/3 -> Bus Creator/2  "LWI_CHECKSUM"
  Read CAN Message/4 -> Bus Creator/3  "LWI_COUNTER"
  Read CAN Message/5 -> Bus Creator/4  "LWI_LWISensorstatus"
  Read CAN Message/6 -> Bus Creator/5  "LWI_LWIQBit_Sub_Daten"
  Read CAN Message/7 -> Write and Read Measurement/1  "LWI_LWIQBit_SteeringWheelAngle"
  Read CAN Message/8 -> Write and Read Measurement1/1  "LWI_LWISteeringWheelAngle"
  Read CAN Message/9 -> Write and Read Measurement2/1  "LWI_LWIVZ_SteeringWheelAngle"
  Read CAN Message/10 -> Write and Read Measurement3/1  "LWI_LWIVZ_SteeringWheelAngle_Speed"
  Read CAN Message/11 -> Write and Read Measurement4/1  "LWI_LWISteeringWheelAngle_Speed"
  Read CAN Message/12 -> Bus Creator/11  "LWI_LWISub_Daten"
  Bus Creator/1 -> Bus Creator2/1, Bus Selector/1  "LWI"
  Write and Read Measurement/1 -> Bus Creator/6  "GOLF_LWIQbit_SteeringWheelAngle"
  Write and Read Measurement1/1 -> Bus Creator/7  "GOLF_LWI_SteeringWheelAngle"
  Write and Read Measurement2/1 -> Bus Creator/8  "GOLF_LWIVZ_SteeringWheelAngle"
  Write and Read Measurement3/1 -> Bus Creator/9  "GOLF_LWIVZ_SteeringWheelAngle_Speed"
  Write and Read Measurement4/1 -> Bus Creator/10  "GOLF_LWI_SteeringWheelAngle_Speed"
  Switch/1 -> Product/1
  Bus Selector/3 -> Switch1/2  "<GOLF_LWIVZ_SteeringWheelAngle_Speed>"
  Write and Read Measurement5/1 -> Bus Creator2/2  "Steering_Angle"
  Constant2/1 -> Switch1/1
  Product1/1 -> Write and Read Measurement6/1
  Bus Selector/2 -> Product/2  "<GOLF_LWI_SteeringWheelAngle>"
  Bus Selector/4 -> Product1/2  "<GOLF_LWI_SteeringWheelAngle_Speed>"
  Constant1/1 -> Switch/3
  Constant3/1 -> Switch1/3
  Switch1/1 -> Product1/1
  Product/1 -> Write and Read Measurement5/1
  Constant/1 -> Switch/1
  Bus Selector/1 -> Switch/2  "<GOLF_LWIVZ_SteeringWheelAngle>"
  Write and Read Measurement6/1 -> Bus Creator2/3  "Steering_Angle_Speed"
  Bus Creator2/1 -> LWI/1

== system Ecotron/Input/Golf/Motor_11 ==
  Bus Creator1 : BusCreator  Inputs=4  OutDataTypeStr=Bus: Msg
      settings: InheritFromInputs=off
  Bus Creator2 : BusCreator  Inputs=3
  Read CAN Message : SF_CanService_Libs/Read CAN Message  typeCAN=Connected  channel=CAN_B  mEn=off  msgInfo=vw_golf  msgItermStore=Motor_11  msgIterm=Motor_11  valid=on  stale=on  motoBit=off  setSignalName=on  flgCustomMonitorVariableRules=on  defineSignalName=off  prefixSignal='rx'  flgValTest=off  flgNoFixed=on  tSample=Task_L1ms  modeCode=Parameterless
  Subsystem1 : Subsystem
  Terminator{,1..4,6..8} (8 alike) : Terminator
  Write and Read Measurement : CoderSF_BSW_Libs/Calibration & Measurement/Write and Read Measurement  variable_name=GOLF_MotorTorque_filtered  variable_value=0  variable_type=single  numD=1  unitStr=""  descStr=""
      settings: AttributesFormatString=type:%<variable_type> Dimensions:%<numD>  SourceProductName=EcoCoder Blocks
  Write and Read Measurement1 : CoderSF_BSW_Libs/Calibration & Measurement/Write and Read Measurement  variable_name=GOLF_MotorTorque_raw  variable_value=0  variable_type=single  numD=1  unitStr=""  descStr=""
      settings: AttributesFormatString=type:%<variable_type> Dimensions:%<numD>  SourceProductName=EcoCoder Blocks
  MatorTorque : Outport
  wires:
  Subsystem1/1("Available ") -> Bus Creator1/1  "Available"
  Bus Creator2/1 -> MatorTorque/1
  Read CAN Message/2 -> Subsystem1/2(Msg_cnt)
  Subsystem1/2(Cnt) -> Bus Creator1/2  "Cnt"
  Read CAN Message/1 -> Subsystem1/1("Available_in ")
  Subsystem1/3(Timeout_Err) -> Bus Creator1/3  "Timeout"
  Bus Creator1/1 -> Bus Creator2/1  "Msg"
  Subsystem1/4(Msg_Freq) -> Bus Creator1/4  "MsgFreq"
  Read CAN Message/9 -> Terminator6/1  "rxMO_MomSchub"
  Read CAN Message/8 -> Write and Read Measurement/1  "rxMO_MomSoll_Filtered"
  Read CAN Message/7 -> Terminator4/1  "rxMO_MomInertia_Total"
  Read CAN Message/6 -> Terminator3/1  "rxMO_MomTotal"
  Read CAN Message/4 -> Terminator1/1  "rxMotor_11BZ"
  Read CAN Message/3 -> Terminator/1  "rxMotor_11CRC"
  Write and Read Measurement/1 -> Bus Creator2/2  "GOLF_MotorTorque_filtered"
  Read CAN Message/12 -> Terminator8/1  "rxMO_QBitMotormomente"
  Read CAN Message/11 -> Terminator7/1  "rxMO_FirstInaccurateThreshold"
  Read CAN Message/10 -> Terminator2/1  "rxMO_StatusNormalOperation_01"
  Read CAN Message/5 -> Write and Read Measurement1/1  "rxMO_MomSoll_Roh"
  Write and Read Measurement1/1 -> Bus Creator2/3  "GOLF_MotorTorque_raw"

== system Ecotron/Input/Golf/Motor_12 ==
  Bus Creator1 : BusCreator  Inputs=4  OutDataTypeStr=Bus: Msg
      settings: InheritFromInputs=off
  Bus Creator2 : BusCreator  Inputs=2
  Read CAN Message : SF_CanService_Libs/Read CAN Message  typeCAN=Connected  channel=CAN_B  mEn=off  msgInfo=vw_golf  msgItermStore=Motor_12  msgIterm=Motor_12  valid=on  stale=on  motoBit=off  setSignalName=on  flgCustomMonitorVariableRules=on  defineSignalName=off  prefixSignal='rx'  flgValTest=off  flgNoFixed=on  tSample=Task_L1ms  modeCode=Parameterless
  Subsystem1 : Subsystem
  Terminator{,1..6} (7 alike) : Terminator
  Write and Read Measurement : CoderSF_BSW_Libs/Calibration & Measurement/Write and Read Measurement  variable_name=GOLF_MotorRPM  variable_value=0  variable_type=single  numD=1  unitStr=""  descStr=""
      settings: AttributesFormatString=type:%<variable_type> Dimensions:%<numD>  SourceProductName=EcoCoder Blocks
  MatorRPM : Outport
  wires:
  Subsystem1/1("Available ") -> Bus Creator1/1  "Available"
  Bus Creator2/1 -> MatorRPM/1
  Read CAN Message/2 -> Subsystem1/2(Msg_cnt)
  Subsystem1/2(Cnt) -> Bus Creator1/2  "Cnt"
  Read CAN Message/1 -> Subsystem1/1("Available_in ")
  Subsystem1/3(Timeout_Err) -> Bus Creator1/3  "Timeout"
  Bus Creator1/1 -> Bus Creator2/1  "Msg"
  Subsystem1/4(Msg_Freq) -> Bus Creator1/4  "MsgFreq"
  Read CAN Message/10 -> Write and Read Measurement/1  "rxMO_RotationSpeed01"
  Read CAN Message/9 -> Terminator6/1  "rxMO_QBitRotationSpeed_01"
  Read CAN Message/8 -> Terminator5/1  "rxMO_Momentenintegral02"
  Read CAN Message/7 -> Terminator4/1  "rxMO_MomLim_dyn"
  Read CAN Message/6 -> Terminator3/1  "rxMO_MomLim_stat"
  Read CAN Message/5 -> Terminator2/1  "rxMO_MomNeg_available"
  Read CAN Message/4 -> Terminator1/1  "rxMotor_12BZ"
  Read CAN Message/3 -> Terminator/1  "rxMotor_12CRC"
  Write and Read Measurement/1 -> Bus Creator2/2  "GOLF_MotorRPM"

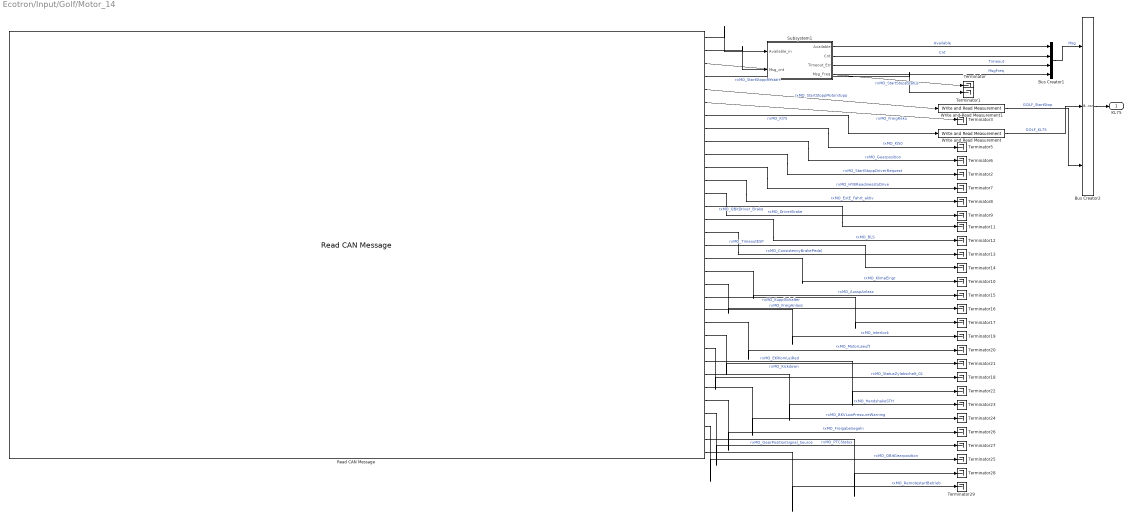
== system Ecotron/Input/Golf/Motor_14 ==
  Bus Creator1 : BusCreator  Inputs=4  OutDataTypeStr=Bus: Msg
      settings: InheritFromInputs=off
  Bus Creator2 : BusCreator  Inputs=3
  Read CAN Message : SF_CanService_Libs/Read CAN Message  typeCAN=Connected  channel=CAN_B  mEn=off  msgInfo=vw_golf  msgItermStore=Motor_14  msgIterm=Motor_14  valid=on  stale=on  motoBit=off  setSignalName=on  flgCustomMonitorVariableRules=on  defineSignalName=off  prefixSignal='rx'  flgValTest=off  flgNoFixed=on  tSample=Task_L1ms  modeCode=Parameterless
  Subsystem1 : Subsystem
  Terminator{,1..3,5..29} (29 alike) : Terminator
  Write and Read Measurement : CoderSF_BSW_Libs/Calibration & Measurement/Write and Read Measurement  variable_name=GOLF_KL75  variable_value=0  variable_type=single  numD=1  unitStr=""  descStr=""
      settings: AttributesFormatString=type:%<variable_type> Dimensions:%<numD>  SourceProductName=EcoCoder Blocks
  Write and Read Measurement1 : CoderSF_BSW_Libs/Calibration & Measurement/Write and Read Measurement  variable_name=GOLF_StartStop  variable_value=0  variable_type=uint8  numD=1  unitStr=""  descStr=""
      settings: AttributesFormatString=type:%<variable_type> Dimensions:%<numD>  SourceProductName=EcoCoder Blocks
  KL75 : Outport
  wires:
  Subsystem1/1("Available ") -> Bus Creator1/1  "Available"
  Bus Creator2/1 -> KL75/1
  Read CAN Message/2 -> Subsystem1/2(Msg_cnt)
  Read CAN Message/7 -> Write and Read Measurement/1  "rxMO_Kl75"
  Subsystem1/2(Cnt) -> Bus Creator1/2  "Cnt"
  Read CAN Message/3 -> Terminator/1  "rxMO_StartStoppStatus"
  Read CAN Message/11 -> Terminator7/1  "rxMO_HYBReadinesstoDrive"
  Read CAN Message/6 -> Terminator3/1  "rxMO_FreigReku"
  Read CAN Message/10 -> Terminator2/1  "rxMO_StartStoppDriverRequest"
  Read CAN Message/1 -> Subsystem1/1("Available_in ")
  Read CAN Message/9 -> Terminator6/1  "rxMO_Gearposition"
  Subsystem1/3(Timeout_Err) -> Bus Creator1/3  "Timeout"
  Bus Creator1/1 -> Bus Creator2/1  "Msg"
  Read CAN Message/13 -> Terminator9/1  "rxMO_DriverBrake"
  Read CAN Message/8 -> Terminator5/1  "rxMO_Kl50"
  Read CAN Message/4 -> Terminator1/1  "rxMO_StartStoppRestart"
  Subsystem1/4(Msg_Freq) -> Bus Creator1/4  "MsgFreq"
  Read CAN Message/12 -> Terminator8/1  "rxMO_ExtE_Fahrt_aktiv"
  Read CAN Message/14 -> Terminator11/1  "rxMO_QBitDriver_Brake"
  Read CAN Message/15 -> Terminator12/1  "rxMO_BLS"
  Read CAN Message/16 -> Terminator13/1  "rxMO_ConsistencyBrakePedal"
  Read CAN Message/17 -> Terminator14/1  "rxMO_TimeoutESP"
  Read CAN Message/18 -> Terminator10/1  "rxMO_KlimaEingr"
  Read CAN Message/19 -> Terminator15/1  "rxMO_AusspAnlass"
  Read CAN Message/20 -> Terminator16/1  "rxMO_FreigAnlass"
  Read CAN Message/21 -> Terminator17/1  "rxMO_KupplSchalter"
  Read CAN Message/22 -> Terminator19/1  "rxMO_Interlock"
  Read CAN Message/23 -> Terminator20/1  "rxMO_MotorLaeuft"
  Read CAN Message/24 -> Terminator21/1  "rxMO_Kickdown"
  Read CAN Message/25 -> Terminator18/1  "rxMO_StatusZylabschalt_01"
  Read CAN Message/26 -> Terminator22/1  "rxMO_EKlKomLeiRed"
  Read CAN Message/27 -> Terminator23/1  "rxMO_HandshakeSTH"
  Read CAN Message/28 -> Terminator24/1  "rxMO_BKVLowPressureWarning"
  Read CAN Message/29 -> Terminator26/1  "rxMO_FreigabeSegeln"
  Read CAN Message/30 -> Terminator27/1  "rxMO_PTCStatus"
  Read CAN Message/31 -> Terminator25/1  "rxMO_QBitGearposition"
  Read CAN Message/32 -> Terminator28/1  "rxMO_GearPositionSignal_Source"
  Read CAN Message/33 -> Terminator29/1  "rxMO_RemotestartBetrieb"
  Read CAN Message/5 -> Write and Read Measurement1/1  "rxMO_StartStoppMotorstopp"
  Write and Read Measurement/1 -> Bus Creator2/2  "GOLF_KL75"
  Write and Read Measurement1/1 -> Bus Creator2/3  "GOLF_StartStop"

== system Ecotron/Input/Golf/Motor_20 ==
  Bus Creator1 : BusCreator  Inputs=4  OutDataTypeStr=Bus: Msg
      settings: InheritFromInputs=off
  Bus Creator2 : BusCreator  Inputs=2
  Read CAN Message : SF_CanService_Libs/Read CAN Message  typeCAN=Connected  channel=CAN_B  mEn=off  msgInfo=vw_golf  msgItermStore=Motor_20  msgIterm=Motor_20  valid=on  stale=on  motoBit=off  setSignalName=on  flgCustomMonitorVariableRules=on  defineSignalName=off  prefixSignal='rx'  flgValTest=off  flgNoFixed=on  tSample=Task_L1ms  modeCode=Parameterless
  Subsystem1 : Subsystem
  Terminator{,1..9} (10 alike) : Terminator
  Write and Read Measurement : CoderSF_BSW_Libs/Calibration & Measurement/Write and Read Measurement  variable_name=GOLF_AcceleratorRawValur  variable_value=0  variable_type=single  numD=1  unitStr=""  descStr=""
      settings: AttributesFormatString=type:%<variable_type> Dimensions:%<numD>  SourceProductName=EcoCoder Blocks
  Accelerator_Pedal : Outport
  wires:
  Read CAN Message/12 -> Terminator8/1  "rxMO_FuelCutOff"
  Subsystem1/4(Msg_Freq) -> Bus Creator1/4  "MsgFreq"
  Read CAN Message/5 -> Write and Read Measurement/1  "rxMO_AcceleratorRawValue01"
  Read CAN Message/4 -> Terminator1/1  "rxCOUNTER"
  Read CAN Message/8 -> Terminator5/1  "rxMO_SigAcceleratorPedalGradient"
  Read CAN Message/13 -> Terminator9/1  "rxMO_TargetSpeed_Idle"
  Bus Creator1/1 -> Bus Creator2/1  "Msg"
  Subsystem1/3(Timeout_Err) -> Bus Creator1/3  "Timeout"
  Read CAN Message/9 -> Terminator6/1  "rxMO_relManifoldPressure"
  Read CAN Message/1 -> Subsystem1/1("Available_in ")
  Read CAN Message/10 -> Terminator2/1  "rxMO_relManifoldPressure_gem_err"
  Read CAN Message/6 -> Terminator3/1  "rxMO_QBitAcceleratorPedalValue_01"
  Read CAN Message/11 -> Terminator7/1  "rxMO_MomentIm_Neutral"
  Read CAN Message/3 -> Terminator/1  "rxCHECKSUM"
  Subsystem1/2(Cnt) -> Bus Creator1/2  "Cnt"
  Read CAN Message/7 -> Terminator4/1  "rxMO_AcceleratorPedalGradient"
  Read CAN Message/2 -> Subsystem1/2(Msg_cnt)
  Bus Creator2/1 -> Accelerator_Pedal/1
  Subsystem1/1("Available ") -> Bus Creator1/1  "Available"
  Write and Read Measurement/1 -> Bus Creator2/2  "GOLF_AcceleratorRawValur"

== system Ecotron/Input/Golf/Subsystem ==
  Bus Creator1 : BusCreator  Inputs=4  OutDataTypeStr=Bus: Msg
      settings: InheritFromInputs=off
  Bus Creator2 : BusCreator  Inputs=2
  Read CAN Message : SF_CanService_Libs/Read CAN Message  typeCAN=Connected  channel=CAN_B  mEn=off  msgInfo=vw_golf  msgItermStore=GearShiftSwitch  msgIterm=GearShiftSwitch  valid=on  stale=on  motoBit=off  setSignalName=on  flgCustomMonitorVariableRules=on  defineSignalName=off  prefixSignal=''  flgValTest=off  flgNoFixed=on  tSample=Task_L1ms  modeCode=Parameterless
  Subsystem1 : Subsystem
  Terminator{1,5..11} (8 alike) : Terminator
  Write and Read Measurement : CoderSF_BSW_Libs/Calibration & Measurement/Write and Read Measurement  variable_name=GOLF_CurrentGear  variable_value=0  variable_type=uint8  numD=1  unitStr=""  descStr=""
      settings: AttributesFormatString=type:%<variable_type> Dimensions:%<numD>  SourceProductName=EcoCoder Blocks
  GearSwitch : Outport
  wires:
  Read CAN Message/4 -> Terminator5/1  "Counter"
  Bus Creator2/1 -> GearSwitch/1
  Read CAN Message/7 -> Terminator7/1  "RandomSignal"
  Read CAN Message/10 -> Terminator10/1  "NoIdea2"
  Read CAN Message/11 -> Terminator11/1  "NoIdea3"
  Read CAN Message/9 -> Terminator9/1  "SwitchRelated2"
  Read CAN Message/8 -> Terminator8/1  "RandomSignal2"
  Read CAN Message/3 -> Terminator1/1  "Checksum"
  Read CAN Message/6 -> Terminator6/1  "SwitchRelated1"
  Subsystem1/2(Cnt) -> Bus Creator1/2  "Cnt"
  Subsystem1/4(Msg_Freq) -> Bus Creator1/4  "MsgFreq"
  Subsystem1/3(Timeout_Err) -> Bus Creator1/3  "Timeout"
  Subsystem1/1("Available ") -> Bus Creator1/1  "Available"
  Read CAN Message/1 -> Subsystem1/1("Available_in ")
  Read CAN Message/2 -> Subsystem1/2(Msg_cnt)
  Bus Creator1/1 -> Bus Creator2/1  "Msg"
  Read CAN Message/5 -> Write and Read Measurement/1  "NoIdea1"
  Write and Read Measurement/1 -> Bus Creator2/2  "GOLF_CurrentGear"

== system Ecotron/Input/Golf/WheelSpeed ==
  Bus Creator : BusCreator  Inputs=5
  Bus Creator1 : BusCreator  Inputs=4  OutDataTypeStr=Bus: Msg
      settings: InheritFromInputs=off
  Read CAN Message : SF_CanService_Libs/Read CAN Message  typeCAN=Connected  channel=CAN_B  mEn=off  msgInfo=vw_golf  msgItermStore=ESP_19  msgIterm=ESP_19  valid=on  stale=on  motoBit=off  setSignalName=on  flgCustomMonitorVariableRules=on  defineSignalName=off  prefixSignal=''  flgValTest=off  flgNoFixed=on  tSample=Task_L1ms  modeCode=Parameterless
  Subsystem1 : Subsystem
  Write and Read Measurement : CoderSF_BSW_Libs/Calibration & Measurement/Write and Read Measurement  variable_name=GOLF_BLWheelSpeed  variable_value=0  variable_type=single  numD=1  unitStr=""  descStr=""
      settings: AttributesFormatString=type:%<variable_type> Dimensions:%<numD>  SourceProductName=EcoCoder Blocks
  Write and Read Measurement1 : CoderSF_BSW_Libs/Calibration & Measurement/Write and Read Measurement  variable_name=GOLF_BRWheelSpeed  variable_value=0  variable_type=single  numD=1  unitStr=""  descStr=""
      settings: AttributesFormatString=type:%<variable_type> Dimensions:%<numD>  SourceProductName=EcoCoder Blocks
  Write and Read Measurement2 : CoderSF_BSW_Libs/Calibration & Measurement/Write and Read Measurement  variable_name=GOLF_FLWheelSpeed  variable_value=0  variable_type=single  numD=1  unitStr=""  descStr=""
      settings: AttributesFormatString=type:%<variable_type> Dimensions:%<numD>  SourceProductName=EcoCoder Blocks
  Write and Read Measurement3 : CoderSF_BSW_Libs/Calibration & Measurement/Write and Read Measurement  variable_name=GOLF_FRWheelSpeed  variable_value=0  variable_type=single  numD=1  unitStr=""  descStr=""
      settings: AttributesFormatString=type:%<variable_type> Dimensions:%<numD>  SourceProductName=EcoCoder Blocks
  "WheelSpeed " : Outport
  wires:
  Read CAN Message/3 -> Write and Read Measurement/1  "ESP_BLWheelSpeed_02"
  Read CAN Message/5 -> Write and Read Measurement2/1  "ESP_FLWheelSpeed_02"
  Read CAN Message/6 -> Write and Read Measurement3/1  "ESP_FRWheelSpeed_02"
  Read CAN Message/4 -> Write and Read Measurement1/1  "ESP_BRWheelSpeed_02"
  Bus Creator/1 -> "WheelSpeed "/1
  Subsystem1/2(Cnt) -> Bus Creator1/2  "Cnt"
  Subsystem1/4(Msg_Freq) -> Bus Creator1/4  "MsgFreq"
  Subsystem1/3(Timeout_Err) -> Bus Creator1/3  "Timeout"
  Subsystem1/1("Available ") -> Bus Creator1/1  "Available"
  Read CAN Message/1 -> Subsystem1/1("Available_in ")
  Read CAN Message/2 -> Subsystem1/2(Msg_cnt)
  Bus Creator1/1 -> Bus Creator/1  "Msg"
  Write and Read Measurement/1 -> Bus Creator/2  "GOLF_BLWheelSpeed"
  Write and Read Measurement1/1 -> Bus Creator/3  "GOLF_BRWheelSpeed"
  Write and Read Measurement2/1 -> Bus Creator/4  "GOLF_FLWheelSpeed"
  Write and Read Measurement3/1 -> Bus Creator/5  "GOLF_FRWheelSpeed"
